simulink model "realimentacao_estados"  (R2020b)
settings: Solver=VariableStepAuto  StartTime=0.0  StopTime=10  RelTol=1e-3
values from neighbouring files (symbols this model uses):
  finalvalue = 1    [script_exp7.m]
  initialvalue = 0    [script_exp7.m]
  K_i = -K(3)    [script_exp7.m]
  K_r = K(1:2)    [script_exp7.m]
  steptime = 0    [script_exp7.m]
undefined symbols (not defined in the file or in its folder): A, B, C, Kt
libraries: simulink x3
settings Model: Creator=gusta  LastModifiedBy=lucas
settings DebuggingCC: SFMachineParentedDataDiag=error

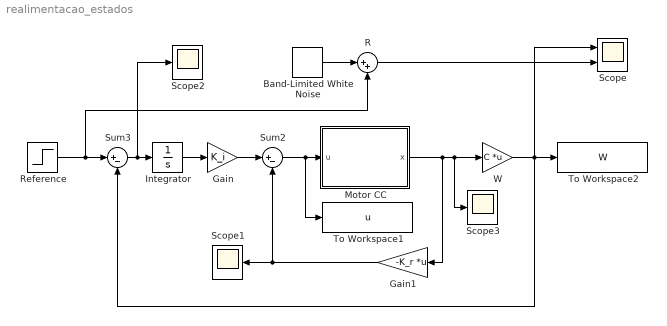
== system realimentacao_estados ==
  Band-Limited White Noise : simulink/Sources/Band-Limited White Noise  Cov=[0.000001]  Ts=0.001  seed=[23341]
  Gain : Gain  Gain=K_i
  Gain1 : Gain  Gain=-K_r  Multiplication=Matrix(K*u)
  Integrator : Integrator
  Motor CC : Subsystem
  R : Sum  Inputs=|++
  Reference : Step  Time=steptime  Before=initialvalue  After=finalvalue  SampleTime=0
  Scope : Scope  NumInputPorts=2
  Scope1 : Scope
  Scope2 : Scope
  Scope3 : Scope
  Sum2 : Sum  Inputs=|+-
  Sum3 : Sum  Inputs=|+-
  To Workspace1 : ToWorkspace  VariableName=u  SaveFormat=Structure With Time  SampleTime=-1
  To Workspace2 : ToWorkspace  VariableName=W  SaveFormat=Structure With Time  SampleTime=-1
  W : Gain  Gain=C  Multiplication=Matrix(K*u)
  wires:
  R/1 -> Scope/2
  Band-Limited White Noise/1 -> R/1
  Reference/1 -> Sum3/1, R/2
  Sum2/1 -> To Workspace1/1, Motor CC/1(u)
  W/1 -> Scope/1, To Workspace2/1, Sum3/2
  Gain1/1 -> Scope1/1, Sum2/2
  Gain/1 -> Sum2/1
  Integrator/1 -> Gain/1
  Sum3/1 -> Scope2/1, Integrator/1
  Motor CC/1(x) -> Gain1/1, Scope3/1, W/1

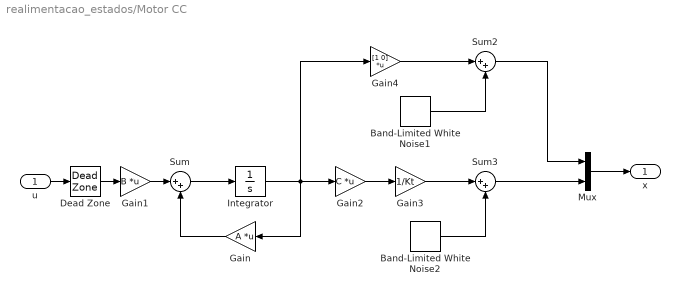
== system realimentacao_estados/Motor CC ==
  u : Inport
  Band-Limited White Noise1 : simulink/Sources/Band-Limited White Noise  Cov=[0.000001]  Ts=0.001  seed=[23341]
  Band-Limited White Noise2 : simulink/Sources/Band-Limited White Noise  Cov=[0.000001]  Ts=0.001  seed=[23341]
  Dead Zone : DeadZone  LowerValue=-3.2  UpperValue=3.2  SaturateOnIntegerOverflow=on
  Gain : Gain  Gain=A  Multiplication=Matrix(K*u)
  Gain1 : Gain  Gain=B  Multiplication=Matrix(K*u)
  Gain2 : Gain  Gain=C  Multiplication=Matrix(K*u)
  Gain3 : Gain  Gain=1/Kt
  Gain4 : Gain  Gain=[1 0]  Multiplication=Matrix(K*u)
  Integrator : Integrator  InitialCondition=[0;0]
  Mux : Mux  Inputs=2
  Sum : Sum  Inputs=|++
  Sum2 : Sum  Inputs=|++
  Sum3 : Sum  Inputs=|++
  x : Outport
  wires:
  Sum/1 -> Integrator/1
  Integrator/1 -> Gain/1, Gain4/1, Gain2/1
  Gain2/1 -> Gain3/1
  Gain1/1 -> Sum/1
  Gain/1 -> Sum/2
  u/1 -> Dead Zone/1
  Dead Zone/1 -> Gain1/1
  Sum2/1 -> Mux/1
  Gain4/1 -> Sum2/1
  Sum3/1 -> Mux/2
  Band-Limited White Noise1/1 -> Sum2/2
  Band-Limited White Noise2/1 -> Sum3/2
  Gain3/1 -> Sum3/1
  Mux/1 -> x/1
